simulink model "preprojeto1simulink"  (R2022a)
settings: Solver=FixedStepAuto  StartTime=0.0  StopTime=10.0  FixedStep=0.001  RelTol=1e-3
settings Model: Creator=a2207206  LastModifiedBy=a2207206

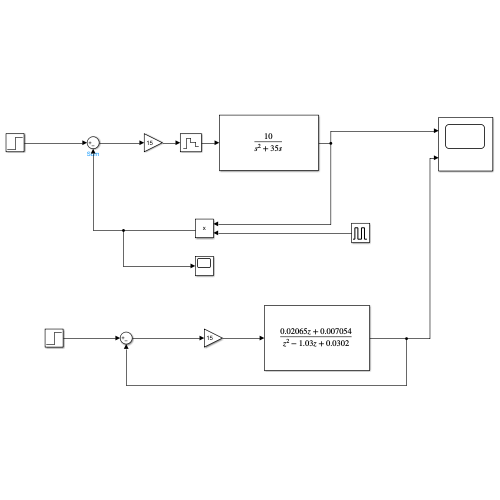
[thumbnail: Simulink's stored preview of the top-level diagram]
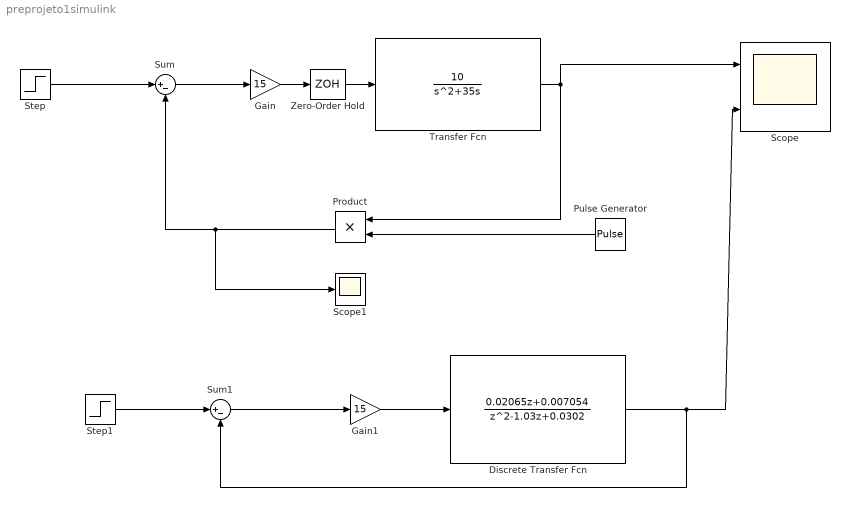
== system preprojeto1simulink ==
  Discrete Transfer Fcn : DiscreteTransferFcn  Numerator=[0.02065 0.007054]  Denominator=[1 -1.03 0.0302]  SampleTime=0.1
  Gain : Gain  Gain=15
  Gain1 : Gain  Gain=15
  Product : Product
  Pulse Generator : DiscretePulseGenerator  PulseType=Time based  Period=0.1
  Scope : Scope  NumInputPorts=2
  Scope1 : Scope
  Step : Step  SampleTime=0
  Step1 : Step  SampleTime=0
  Sum : Sum  Inputs=|+-
  Sum1 : Sum  Inputs=|+-
  Transfer Fcn : TransferFcn  Numerator=[10]  Denominator=[1 35 0]
  Zero-Order Hold : ZeroOrderHold  SampleTime=0.1
  wires:
  Sum/1 -> Gain/1
  Transfer Fcn/1 -> Product/1, Scope/1
  Step/1 -> Sum/1
  Pulse Generator/1 -> Product/2
  Product/1 -> Scope1/1, Sum/2
  Gain/1 -> Zero-Order Hold/1
  Zero-Order Hold/1 -> Transfer Fcn/1
  Sum1/1 -> Gain1/1
  Gain1/1 -> Discrete Transfer Fcn/1
  Step1/1 -> Sum1/1
  Discrete Transfer Fcn/1 -> Scope/2, Sum1/2
